simulink model "LW_ctrl_241029_1"  (R2024b)
settings: Solver=ode4  StartTime=0.0  StopTime=inf  FixedStep=0.005  RelTol=1e-3  EnableMultiTasking=on
StartFcn:
  | %timestart = cputime;
StopFcn:
  | %dt = cputime - timestart
undefined symbols (not defined in the file or in its folder): AttCtrl_cycle, ControlMode, DEG2RAD, Earth, FlightMode, LW_ACRO_P_MAX, LW_ACRO_R_MAX, LW_ACRO_Y_MAX, LW_AERO_C0, LW_AERO_C1, LW_AERO_Y0, LW_ANGLE, LW_DMZ0, LW_DMZ_MIN, LW_LAT_CIRCLE, LW_MAN_PITCH_MAX, LW_MAN_ROLL_MAX, LW_MASS, LW_OB_CIRCLE_R, LW_OB_CIRCLE_V, LW_OB_CIRCLE_W, LW_OB_TYPE, LW_REX_YAW, LW_SERVOL_MAX, LW_SERVOR_MAX, LW_TEST_DTXY, LW_TEST_DTZ, LW_THR_HOVER, LW_WZ_MAX, LW_X_ACCEL_MAX, LW_X_ACCEL_MIN, LW_X_FF, LW_X_JERK_MAX, LW_X_P, LW_X_VEL_MAX, LW_Y_ACCEL_MAX, LW_Y_ACCEL_MIN, LW_Y_FF, LW_Y_JERK_MAX, LW_Y_P, LW_Y_VEL_MAX, LW_YAW_KAD, LW_YAW_KAP, LW_Z_ACCEL_LOW, LW_Z_ACCEL_UP, LW_Z_FF, LW_Z_JERK_MAX, LW_Z_P, LW_Z_VEL_MAX_UP, Map_xoffset, Map_yoffset, Map_zoffset, MAX_wdotx, MAX_wdoty, MAX_wdotz, Mixer_cycle, ModelParam_AccelMax, ModelParam_DelayAtt, ModelParam_DelayOmega, ModelParam_DelayPos ... (+59)
libraries: pixhawk_slib_uORB_RW x15, simulink x7, slpidlib x6, dspfdesign x6, dspstat3 x5, aerolibnav x4, pixhawk_slib_sensors_actuators x3, aerolibtransform2 x3, etargetslib x2, pixhawk_slib_rfly x1, aerolibatmos2 x1, slrealtimeiplib x1
(part 6 of 6)

== matlab function LW_ctrl_241029_1/states_update/vehicle_local_position/HIL&FLY V1.13.3/DisturbanceEstimator ==
  data: Va input; qm input single; omegam input single; T input single; ModelParam_uavJ parameter; ModelParam_motorJm parameter; ModelParam_rotorEta parameter; ModelParam_rotordx parameter; ModelParam_rotordy parameter; ModelParam_rotorCm parameter; ModelParam_rotorCt parameter; qk_ output; omegak_ output; d_hat output single size=[3,1]; LW_TEST_WNXY parameter; LW_TEST_WNZ parameter; LW_TEST_LAMXY parameter; LW_TEST_LAMZ parameter; LW_TEST_SIGXY parameter; LW_TEST_SIGZ parameter; ModelParam_LBb parameter; ModelParam_LBc parameter; ModelParam_LBS parameter; LW_ANGLE parameter; ModelParam_LBRho parameter; LW_USE_SER parameter; LW_LBCL_D parameter; LW_LBCM_D parameter; ModelParam_LBCn_d parameter; LW_TEST_TDT parameter; quat_reset_counter input; delta_q_reset input; dt input single
function [qk_, omegak_, d_hat] = DisturbanceEstimator(Va, qm, omegam, T,...
    ModelParam_uavJ,ModelParam_motorJm, ModelParam_rotorEta, ModelParam_rotordx, ModelParam_rotordy, ModelParam_rotorCm, ModelParam_rotorCt,...
    LW_TEST_WNXY, LW_TEST_WNZ,LW_TEST_LAMXY, LW_TEST_LAMZ, LW_TEST_SIGXY, LW_TEST_SIGZ, ModelParam_LBb, ModelParam_LBc, ModelParam_LBS, LW_ANGLE, ...
    ModelParam_LBRho, LW_USE_SER, LW_LBCL_D, LW_LBCM_D, ModelParam_LBCn_d, LW_TEST_TDT, quat_reset_counter, delta_q_reset, dt)

persistent tau_qk tau_omegak tau_z3
persistent  quat_reset_counter_
if isempty(quat_reset_counter_)
    quat_reset_counter_ = quat_reset_counter;
end

if isInfNan(qm)
    qm = single([1;0;0;0]);
else
    %qm = qm/(sqrt(qm'*qm));
    %qm = quatnormalize(qm');
    qm = qm(:);
end
if isInfNan(omegam)
    omegam = single([0;0;0]);
else
    omegam = omegam(:);
end
if isInfNan(T)
    T = single([0;0;0;0;0;0]);
else
    T = T(:);
end
if dt < 0.001
    dt = single(0.001);
elseif dt > 0.02
    dt = single(0.02);
end

if isempty(tau_qk)
    if notInfNan(qm)
        tau_qk = qm;
    else
        tau_qk = single([1;0;0;0]);
    end
end
if isInfNan(tau_qk)
    if notInfNan(qm)
        tau_qk = qm;
    else
        tau_qk = single([1;0;0;0]);
    end
end
if isempty(tau_omegak)
    if notInfNan(omegam)
        tau_omegak = omegam;
    else
        tau_omegak = single([0;0;0]);
    end
end
if isInfNan(tau_omegak)
    if notInfNan(omegam)
        tau_omegak = omegam;
    else
        tau_omegak = single([0;0;0]);
    end
end
if isempty(tau_z3)
    tau_z3 = single([0;0;0]);
end
if isInfNan(tau_z3)
    tau_z3 = single([0;0;0]);
end



%结构参数
rotorEta = single(ModelParam_rotorEta);
rotordx = single(ModelParam_rotordx);
rotordy = single(ModelParam_rotordy);
LBb = single(ModelParam_LBb);
LBc = single(ModelParam_LBc);
LBS = single(ModelParam_LBS);
kappa = single(LW_ANGLE*pi/180);
Rho = single(ModelParam_LBRho);
%动力系统参数
rotorCm = single(ModelParam_rotorCm);
rotorCt = single(ModelParam_rotorCt);
km_f = rotorCm/rotorCt;
Cl_d = single(LW_LBCL_D);
Cm_d = single(LW_LBCM_D);
Cn_d = single(ModelParam_LBCn_d);
%
Va_ = max(Va,0.1);
if LW_USE_SER > 0.5
    Q = 0.5*Rho*Va_^2*LBS;
else
    Q = single(0);
end
%滤波器参数
L = eye(3,2,"single");
wn = [LW_TEST_WNXY;LW_TEST_WNXY;LW_TEST_WNZ];%rad/s
sigma = [LW_TEST_SIGXY;LW_TEST_SIGXY;LW_TEST_SIGZ];
L(:,1) = wn.^2;
L(:,2) = 2*sigma.*wn;
lamda = single([LW_TEST_LAMXY;LW_TEST_LAMXY;LW_TEST_LAMZ]);
%滤波器结构
%reset处理
if quat_reset_counter_ ~= quat_reset_counter
    tau_q = quatmultiply(delta_q_reset(:)',tau_qk');
    tau_qk = tau_q';
    quat_reset_counter_ = quat_reset_counter;
end
q_err = quatmultiply(quatconj(tau_qk'), qm');
q_err = quatnormalize(q_err);
eta = constrain(q_err(1), single(-1), single(1));
epsilon = q_err(2 : 4);
theta = 2 * acos(eta);
theta = wrap_pi(theta);
if abs(theta) < 0.0873 % 5*pi/180
    Xi_e = sign(eta) * 2 * epsilon;
else
    Xi_e = sign(eta) / sin(theta / 2) * theta * epsilon;
end
e_q = Xi_e(:);
e_omega = omegam - tau_omegak;

%inv_uavJ = eye(3,3)/ModelParam_uavJ;
inv_uavJ = eye(3);
for ii = 1:3
    inv_uavJ(ii,ii) = 1/(ModelParam_uavJ(ii,ii));
end
%le = l1*eq+l2*ew
Le = L(:,1).*e_q + L(:,2).*e_omega;
K1 = km_f;
coseta = cos(rotorEta);
K2 = rotordy*coseta;
dxcoseta = rotordx*coseta;
%估计螺旋桨推力，根据混控器输出滤波得到
T = LowPass(T, LW_TEST_TDT);
B = [-K2       -K2        K2       K2      -Q*LBb*Cl_d*cos(kappa) Q*LBb*Cl_d*cos(kappa);
     dxcoseta  -dxcoseta dxcoseta -dxcoseta Q*LBc*Cm_d Q*LBc*Cm_d;
     K1        -K1       -K1      K1      Q*LBb*Cl_d*sin(kappa) -Q*LBb*Cl_d*sin(kappa)];
z3_ = tau_z3 + lamda.*Le*dt;
if LW_USE_SER > 0.5
    Fr = B*T;
else
    Fr = B(:,1:4)*T(1:4);
end

omegak_ = tau_omegak +(Le + z3_ + inv_uavJ*Fr- inv_uavJ*(cross(omegam,ModelParam_uavJ*omegam)))*dt;
delta_theta = [0 -omegak_(1) -omegak_(2) -omegak_(3);
               omegak_(1) 0 omegak_(3) -omegak_(2);
               omegak_(2) -omegak_(3) 0 omegak_(1);
               omegak_(3) omegak_(2) -omegak_(1) 0]*dt;
qk_ = (eye(4) + delta_theta/2)*tau_qk;
qk_ = qk_/(sqrt(qk_'*qk_));
d_hat = ModelParam_uavJ*(Le + z3_);

if notInfNan(z3_) && notInfNan(omegak_) && notInfNan(qk_)
    tau_z3 = z3_;
    tau_omegak = omegak_;
    tau_qk = qk_;
else
    tau_z3 = single([0;0;0]);
    tau_omegak = omegam;
    tau_qk = qm;
end

end

function d_est = LowPass(d_est,DT)
% DT = dt/(dt + Ts)
% 其中dt是采样周期，Ts是低通滤波器的时间常数
% 截止频率f = 1/Ts/2pi Hz
% 如 dt=0.004, f=30Hz , LW_TEST_DT=0.43
persistent d_est_last
if isempty(d_est_last)
    d_est_last = d_est;
end
if isInfNan(d_est_last)
    d_est_last = zeros(size(d_est),'single');
end
d_est = d_est_last + DT*(d_est - d_est_last);
d_est_last = d_est;
end

== matlab function LW_ctrl_241029_1/rc_receive/manual_ctrl_in/Sim/Simulate RC/InputConditioning/deadzone1 ==
  data: u input; y output; rc_min input; rc_max input
function y = fcn(u, rc_min, rc_max)
%Function description:
%  Control the range of the remote control input from RCMin to RCMax, and set
%  a dead zone with a dead zone size of ±deadZone,the output y is
%  normalized to 0~1.You can get the RC calibration parameters in QGC.
RCMin = rc_min;
RCMax = rc_max;
RCMid = ((RCMin + RCMax)/2);
deadZoneRate = double(0.05);
deadZone = deadZoneRate*(RCMax - RCMin);
k = 1/(RCMax - RCMid - deadZone);
%Limiting
if(u < RCMin)
    u = RCMin;
elseif(u > RCMax)
    u = RCMax;
end
%dead zone and normalize
 if(u > RCMid + deadZone)
    y = single((u-RCMid - deadZone)*k);
 elseif(u < RCMid - deadZone)
     y = single((u - RCMid + deadZone)*k);
 else
     y = single(0);
 end
 end

== matlab function LW_ctrl_241029_1/navigator/logger/HIL&FLY/hrt_timestamp ==
  data: ts output
function ts  = fcn
% coder.cinclude('drivers/drv_hrt.h');
persistent count
if isempty(count)
    count = 0;
end

hrt = 0;
if coder.target('Rtw')
    hrt = coder.ceval('hrt_absolute_time');
else
    hrt = count;
end
ts = hrt;% us

count = count + 1;

== matlab function LW_ctrl_241029_1/rc_receive/manual_ctrl_in/Sim/Simulate RC/InputConditioning/deadzone2 ==
  data: u input; y output; rc_min input; rc_max input
function y = fcn(u, rc_min, rc_max)
%Function description:
%  Control the range of the remote control input from RCMin to RCMax, and set
%  a dead zone with a dead zone size of ±deadZone,the output y is
%  normalized to 0~1.You can get the RC calibration parameters in QGC.
RCMin = rc_min;
RCMax = rc_max;
RCMid = ((RCMin + RCMax)/2);
deadZoneRate = double(0.05);
deadZone = deadZoneRate*(RCMax - RCMin);
k = 1/(RCMax - RCMid - deadZone);
%Limiting
if(u < RCMin)
    u = RCMin;
elseif(u > RCMax)
    u = RCMax;
end
%dead zone and normalize
 if(u > RCMid + deadZone)
    y = single((u-RCMid - deadZone)*k);
 elseif(u < RCMid - deadZone)
     y = single((u - RCMid + deadZone)*k);
 else
     y = single(0);
 end
 end

== matlab function LW_ctrl_241029_1/state_machine/logger/HIL&FLY/hrt_timestamp ==
  data: ts output
function ts  = fcn
% coder.cinclude('drivers/drv_hrt.h');
persistent count
if isempty(count)
    count = 0;
end

hrt = 0;
if coder.target('Rtw')
    hrt = coder.ceval('hrt_absolute_time');
else
    hrt = count;
end
ts = hrt;% us

count = count + 1;

== matlab function LW_ctrl_241029_1/rc_receive/manual_ctrl_in/HIL&FLY V1.13.3/logger/hrt_timestamp ==
  data: ts output
function ts  = fcn
% coder.cinclude('drivers/drv_hrt.h');
persistent count
if isempty(count)
    count = 0;
end

hrt = 0;
if coder.target('Rtw')
    hrt = coder.ceval('hrt_absolute_time');
else
    hrt = count;
end
ts = hrt;% us

count = count + 1;

== matlab function LW_ctrl_241029_1/rc_receive/manual_ctrl_in/Sim/Simulate RC/InputConditioning/deadzone3 ==
  data: u input; y output; rc_min input; rc_max input
function y = fcn(u, rc_min, rc_max)
%Function description:
%  Control the range of the remote control input from RCMin to RCMax, and set
%  a dead zone with a dead zone size of ±deadZone,the output y is
%  normalized to 0~1.You can get the RC calibration parameters in QGC.
RCMin = rc_min;
RCMax = rc_max;
RCMid = ((RCMin + RCMax)/2);
deadZoneRate = double(0.05);
deadZone = deadZoneRate*(RCMax - RCMin);
k = 1/(RCMax - RCMid - deadZone);
%Limiting
if(u < RCMin)
    u = RCMin;
elseif(u > RCMax)
    u = RCMax;
end
%dead zone and normalize
 if(u > RCMid + deadZone)
    y = single((u-RCMid - deadZone)*k);
 elseif(u < RCMid - deadZone)
     y = single((u - RCMid + deadZone)*k);
 else
     y = single(0);
 end
 end

== matlab function LW_ctrl_241029_1/states_update/vehicle_local_position/Sim/nan_inf_q ==
  data: u input; y output
function y = fcn(u)

for i = 1:length(u)
    if isnan(u(i)) || isinf(u(i))
        if i == 1
            u(i) = single(1);
        else
            u(i) = single(0);
        end
    end
end
y = u;

== matlab function LW_ctrl_241029_1/navigator/navigator_manual/roll_deadzone ==
  data: u input; y output; LW_MAN_ROLL_DZ parameter
function y = fcn(u, LW_MAN_ROLL_DZ)
%Function description:
%  set a dead zone with a dead zone size of ±deadZone.
RCMin = single(-1);
RCMax = single(1);
RCMid = ((RCMin + RCMax)/2);
deadZone = LW_MAN_ROLL_DZ;
k = 1/(RCMax - RCMid - deadZone);

%dead zone
if(u > RCMid + deadZone)
    y = single((u-RCMid - deadZone)*k);
elseif(u < RCMid - deadZone)
    y = single((u - RCMid + deadZone)*k);
else
    y = single(0);
end
end

== matlab function LW_ctrl_241029_1/navigator/navigator_manual/pitch_deadzone ==
  data: u input; y output; LW_MAN_PITCH_DZ parameter
function y = fcn(u, LW_MAN_PITCH_DZ)
%Function description:
%  set a dead zone with a dead zone size of ±deadZone.
RCMin = single(-1);
RCMax = single(1);
RCMid = ((RCMin + RCMax)/2);
deadZone = LW_MAN_PITCH_DZ;
k = 1/(RCMax - RCMid - deadZone);

%dead zone
if(u > RCMid + deadZone)
    y = single((u-RCMid - deadZone)*k);
elseif(u < RCMid - deadZone)
    y = single((u - RCMid + deadZone)*k);
else
    y = single(0);
end
end

== matlab function LW_ctrl_241029_1/navigator/navigator_manual/rollrate_deadzone ==
  data: u input; y output; LW_MAN_WX_DZ parameter
function y = fcn(u, LW_MAN_WX_DZ)
%Function description:
%  set a dead zone with a dead zone size of ±deadZone.
RCMin = single(-1);
RCMax = single(1);
RCMid = ((RCMin + RCMax)/2);
deadZone = LW_MAN_WX_DZ;
k = 1/(RCMax - RCMid - deadZone);

%dead zone
if(u > RCMid + deadZone)
    y = single((u-RCMid - deadZone)*k);
elseif(u < RCMid - deadZone)
    y = single((u - RCMid + deadZone)*k);
else
    y = single(0);
end
end

== matlab function LW_ctrl_241029_1/navigator/navigator_manual/pitchrate_deadzone ==
  data: u input; y output; LW_MAN_WY_DZ parameter
function y = fcn(u, LW_MAN_WY_DZ)
%Function description:
%  set a dead zone with a dead zone size of ±deadZone.
RCMin = single(-1);
RCMax = single(1);
RCMid = ((RCMin + RCMax)/2);
deadZone = LW_MAN_WY_DZ;
k = 1/(RCMax - RCMid - deadZone);

%dead zone
if(u > RCMid + deadZone)
    y = single((u-RCMid - deadZone)*k);
elseif(u < RCMid - deadZone)
    y = single((u - RCMid + deadZone)*k);
else
    y = single(0);
end
end

== matlab function LW_ctrl_241029_1/navigator/navigator_manual/yawrate_deadzone ==
  data: u input; y output; LW_MAN_WZ_DZ parameter
function y = fcn(u, LW_MAN_WZ_DZ)
%Function description:
%  set a dead zone with a dead zone size of ±deadZone.
RCMin = single(-1);
RCMax = single(1);
RCMid = ((RCMin + RCMax)/2);
deadZone = LW_MAN_WZ_DZ;
k = 1/(RCMax - RCMid - deadZone);

%dead zone
if(u > RCMid + deadZone)
    y = single((u-RCMid - deadZone)*k);
elseif(u < RCMid - deadZone)
    y = single((u - RCMid + deadZone)*k);
else
    y = single(0);
end
end

== matlab function LW_ctrl_241029_1/navigator/navigator_manual/vx_deadzone ==
  data: u input; y output; LW_X_VEL_DZ parameter
function y = fcn(u, LW_X_VEL_DZ)
%Function description:
%  set a dead zone with a dead zone size of ±deadZone.
RCMin = single(-1);
RCMax = single(1);
RCMid = ((RCMin + RCMax)/2);
deadZone = LW_X_VEL_DZ;
k = 1/(RCMax - RCMid - deadZone);

%dead zone
if(u > RCMid + deadZone)
    y = single((u-RCMid - deadZone)*k);
elseif(u < RCMid - deadZone)
    y = single((u - RCMid + deadZone)*k);
else
    y = single(0);
end
end

== matlab function LW_ctrl_241029_1/navigator/navigator_manual/vy_deadzone ==
  data: u input; y output; LW_Y_VEL_DZ parameter
function y = fcn(u, LW_Y_VEL_DZ)
%Function description:
%  set a dead zone with a dead zone size of ±deadZone.
RCMin = single(-1);
RCMax = single(1);
RCMid = ((RCMin + RCMax)/2);
deadZone = LW_Y_VEL_DZ;
k = 1/(RCMax - RCMid - deadZone);

%dead zone
if(u > RCMid + deadZone)
    y = single((u-RCMid - deadZone)*k);
elseif(u < RCMid - deadZone)
    y = single((u - RCMid + deadZone)*k);
else
    y = single(0);
end
end

== matlab function LW_ctrl_241029_1/navigator/navigator_manual/vz_deadzone ==
  data: u input; y output; LW_Z_VEL_DZ parameter
function y = fcn(u, LW_Z_VEL_DZ)
%Function description:
%  set a dead zone with a dead zone size of ±deadZone.
% u:0-1
u = u*2 - 1; % -1~1
RCMin = single(-1);
RCMax = single(1);
RCMid = ((RCMin + RCMax)/2);
deadZone = LW_Z_VEL_DZ;
k = 1/(RCMax - RCMid - deadZone);

%dead zone
if(u > RCMid + deadZone)
    y = single((u-RCMid - deadZone)*k);
elseif(u < RCMid - deadZone)
    y = single((u - RCMid + deadZone)*k);
else
    y = single(0);
end
end

== matlab function LW_ctrl_241029_1/rc_receive/manual_ctrl_in/Sim/Simulate ref/commandMapping/command2pwm/stabilized/roll_deadzone_inv ==
  data: u input; y output; LW_MAN_ROLL_DZ parameter
function y = fcn(u, LW_MAN_ROLL_DZ)
%Function description:
%  set a dead zone with a dead zone size of ±deadZone.
RCMin = single(-1);
RCMax = single(1);
RCMid = ((RCMin + RCMax)/2);
deadZone = LW_MAN_ROLL_DZ;
k = 1/(RCMax - RCMid - deadZone);

%dead zone
if(u > RCMid + deadZone)
    y = single(u/k + RCMid + deadZone);
elseif(u < RCMid - deadZone)
     y = single(u/k + RCMid - deadZone);
else
    y = single(0);
end
end

== matlab function LW_ctrl_241029_1/rc_receive/manual_ctrl_in/Sim/Simulate ref/commandMapping/command2pwm/stabilized/pitch_deadzone_inv ==
  data: u input; y output; LW_MAN_PITCH_DZ parameter
function y = fcn(u, LW_MAN_PITCH_DZ)
%Function description:
%  set a dead zone with a dead zone size of ±deadZone.
RCMin = single(-1);
RCMax = single(1);
RCMid = ((RCMin + RCMax)/2);
deadZone = LW_MAN_PITCH_DZ;
k = 1/(RCMax - RCMid - deadZone);

%dead zone
if(u > RCMid + deadZone)
    y = single(u/k + RCMid + deadZone);
elseif(u < RCMid - deadZone)
     y = single(u/k + RCMid - deadZone);
else
    y = single(0);
end
end

== matlab function LW_ctrl_241029_1/rc_receive/manual_ctrl_in/Sim/Simulate ref/commandMapping/command2pwm/stabilized/yawrare_deadzone_inv ==
  data: u input; y output; LW_MAN_WZ_DZ parameter
function y = fcn(u, LW_MAN_WZ_DZ)
%Function description:
%  set a dead zone with a dead zone size of ±deadZone.
RCMin = single(-1);
RCMax = single(1);
RCMid = ((RCMin + RCMax)/2);
deadZone = LW_MAN_WZ_DZ;
k = 1/(RCMax - RCMid - deadZone);

%dead zone
if(u > RCMid + deadZone)
    y = single(u/k + RCMid + deadZone);
elseif(u < RCMid - deadZone)
     y = single(u/k + RCMid - deadZone);
else
    y = single(0);
end
end

== matlab function LW_ctrl_241029_1/rc_receive/manual_ctrl_in/Sim/Simulate ref/commandMapping/command2pwm/altitude/pitch_deadzone_inv ==
  data: u input; y output; LW_MAN_PITCH_DZ parameter
function y = fcn(u, LW_MAN_PITCH_DZ)
%Function description:
%  set a dead zone with a dead zone size of ±deadZone.
RCMin = single(-1);
RCMax = single(1);
RCMid = ((RCMin + RCMax)/2);
deadZone = LW_MAN_PITCH_DZ;
k = 1/(RCMax - RCMid - deadZone);

%dead zone
if(u > RCMid + deadZone)
    y = single(u/k + RCMid + deadZone);
elseif(u < RCMid - deadZone)
     y = single(u/k + RCMid - deadZone);
else
    y = single(0);
end
end

== matlab function LW_ctrl_241029_1/rc_receive/manual_ctrl_in/Sim/Simulate ref/commandMapping/command2pwm/altitude/roll_deadzone_inv ==
  data: u input; y output; LW_MAN_ROLL_DZ parameter
function y = fcn(u, LW_MAN_ROLL_DZ)
%Function description:
%  set a dead zone with a dead zone size of ±deadZone.
RCMin = single(-1);
RCMax = single(1);
RCMid = ((RCMin + RCMax)/2);
deadZone = LW_MAN_ROLL_DZ;
k = 1/(RCMax - RCMid - deadZone);

%dead zone
if(u > RCMid + deadZone)
    y = single(u/k + RCMid + deadZone);
elseif(u < RCMid - deadZone)
     y = single(u/k + RCMid - deadZone);
else
    y = single(0);
end
end

== matlab function LW_ctrl_241029_1/rc_receive/manual_ctrl_in/Sim/Simulate ref/commandMapping/command2pwm/acro/wz_deadzone_inv ==
  data: u input; y output; LW_MAN_WZ_DZ parameter
function y = fcn(u, LW_MAN_WZ_DZ)
%Function description:
%  set a dead zone with a dead zone size of ±deadZone.
RCMin = single(-1);
RCMax = single(1);
RCMid = ((RCMin + RCMax)/2);
deadZone = LW_MAN_WZ_DZ;
k = 1/(RCMax - RCMid - deadZone);

%dead zone
if(u > RCMid + deadZone)
    y = single(u/k + RCMid + deadZone);
elseif(u < RCMid - deadZone)
     y = single(u/k + RCMid - deadZone);
else
    y = single(0);
end
end

== matlab function LW_ctrl_241029_1/rc_receive/manual_ctrl_in/Sim/Simulate ref/commandMapping/command2pwm/acro/wx_deadzone_inv ==
  data: u input; y output; LW_MAN_WX_DZ parameter
function y = fcn(u, LW_MAN_WX_DZ)
%Function description:
%  set a dead zone with a dead zone size of ±deadZone.
RCMin = single(-1);
RCMax = single(1);
RCMid = ((RCMin + RCMax)/2);
deadZone = LW_MAN_WX_DZ;
k = 1/(RCMax - RCMid - deadZone);

%dead zone
if(u > RCMid + deadZone)
    y = single(u/k + RCMid + deadZone);
elseif(u < RCMid - deadZone)
     y = single(u/k + RCMid - deadZone);
else
    y = single(0);
end
end

== matlab function LW_ctrl_241029_1/rc_receive/manual_ctrl_in/Sim/Simulate ref/commandMapping/command2pwm/acro/wy_deadzone_inv ==
  data: u input; y output; LW_MAN_WY_DZ parameter
function y = fcn(u, LW_MAN_WY_DZ)
%Function description:
%  set a dead zone with a dead zone size of ±deadZone.
RCMin = single(-1);
RCMax = single(1);
RCMid = ((RCMin + RCMax)/2);
deadZone = LW_MAN_WY_DZ;
k = 1/(RCMax - RCMid - deadZone);

%dead zone
if(u > RCMid + deadZone)
    y = single(u/k + RCMid + deadZone);
elseif(u < RCMid - deadZone)
     y = single(u/k + RCMid - deadZone);
else
    y = single(0);
end
end

== matlab function LW_ctrl_241029_1/rc_receive/manual_ctrl_in/Sim/Simulate ref/commandMapping/command2pwm/position/wz_deadzone_inv ==
  data: u input; y output; LW_MAN_WZ_DZ parameter
function y = fcn(u, LW_MAN_WZ_DZ)
%Function description:
%  set a dead zone with a dead zone size of ±deadZone.
RCMin = single(-1);
RCMax = single(1);
RCMid = ((RCMin + RCMax)/2);
deadZone = LW_MAN_WZ_DZ;
k = 1/(RCMax - RCMid - deadZone);

%dead zone
if(u > RCMid + deadZone)
    y = single(u/k + RCMid + deadZone);
elseif(u < RCMid - deadZone)
     y = single(u/k + RCMid - deadZone);
else
    y = single(0);
end
end

== matlab function LW_ctrl_241029_1/rc_receive/manual_ctrl_in/Sim/Simulate ref/commandMapping/command2pwm/position/vz_deadzone_inv ==
  data: u input; y output; LW_Z_VEL_DZ parameter
function y = fcn(u, LW_Z_VEL_DZ)
%Function description:
%  set a dead zone with a dead zone size of ±deadZone.
RCMin = single(-1);
RCMax = single(1);
RCMid = ((RCMin + RCMax)/2);
deadZone = LW_Z_VEL_DZ;
k = 1/(RCMax - RCMid - deadZone);

%dead zone
if(u > RCMid + deadZone)
    y = single(u/k + RCMid + deadZone);
elseif(u < RCMid - deadZone)
     y = single(u/k + RCMid - deadZone);
else
    y = single(0);
end

y = (y+1)*0.5;
end

== matlab function LW_ctrl_241029_1/rc_receive/manual_ctrl_in/Sim/Simulate ref/commandMapping/command2pwm/position/vy_deadzone_inv ==
  data: u input; y output; LW_Y_VEL_DZ parameter
function y = fcn(u, LW_Y_VEL_DZ)
%Function description:
%  set a dead zone with a dead zone size of ±deadZone.
RCMin = single(-1);
RCMax = single(1);
RCMid = ((RCMin + RCMax)/2);
deadZone = LW_Y_VEL_DZ;
k = 1/(RCMax - RCMid - deadZone);

%dead zone
if(u > RCMid + deadZone)
    y = single(u/k + RCMid + deadZone);
elseif(u < RCMid - deadZone)
     y = single(u/k + RCMid - deadZone);
else
    y = single(0);
end
end

== matlab function LW_ctrl_241029_1/rc_receive/manual_ctrl_in/Sim/Simulate ref/commandMapping/command2pwm/position/vx_deadzone_inv ==
  data: u input; y output; LW_X_VEL_DZ parameter
function y = fcn(u, LW_X_VEL_DZ)
%Function description:
%  set a dead zone with a dead zone size of ±deadZone.
RCMin = single(-1);
RCMax = single(1);
RCMid = ((RCMin + RCMax)/2);
deadZone = LW_X_VEL_DZ;
k = 1/(RCMax - RCMid - deadZone);

%dead zone
if(u > RCMid + deadZone)
    y = single(u/k + RCMid + deadZone);
elseif(u < RCMid - deadZone)
     y = single(u/k + RCMid - deadZone);
else
    y = single(0);
end
end

== matlab function LW_ctrl_241029_1/rc_receive/manual_ctrl_in/Sim/Simulate ref/commandMapping/command2pwm/altitude/vz_deadzone_inv ==
  data: u input; y output; LW_Z_VEL_DZ parameter
function y = fcn(u, LW_Z_VEL_DZ)
%Function description:
%  set a dead zone with a dead zone size of ±deadZone.
RCMin = single(-1);
RCMax = single(1);
RCMid = ((RCMin + RCMax)/2);
deadZone = LW_Z_VEL_DZ;
k = 1/(RCMax - RCMid - deadZone);

%dead zone
if(u > RCMid + deadZone)
    y = single(u/k + RCMid + deadZone);
elseif(u < RCMid - deadZone)
     y = single(u/k + RCMid - deadZone);
else
    y = single(0);
end

y = (y+1)*0.5;
end

== matlab function LW_ctrl_241029_1/rc_receive/manual_ctrl_in/Sim/Simulate ref/commandMapping/command2pwm/altitude/wz_deadzone_inv ==
  data: u input; y output; LW_MAN_WZ_DZ parameter
function y = fcn(u, LW_MAN_WZ_DZ)
%Function description:
%  set a dead zone with a dead zone size of ±deadZone.
RCMin = single(-1);
RCMax = single(1);
RCMid = ((RCMin + RCMax)/2);
deadZone = LW_MAN_WZ_DZ;
k = 1/(RCMax - RCMid - deadZone);

%dead zone
if(u > RCMid + deadZone)
    y = single(u/k + RCMid + deadZone);
elseif(u < RCMid - deadZone)
     y = single(u/k + RCMid - deadZone);
else
    y = single(0);
end
end

== matlab function LW_ctrl_241029_1/states_update/vehicle_local_position/Sim/getIncid ==
  data: q input; incid output; LW_ANGLE parameter
function incid = fcn(q, LW_ANGLE)

if notInfNan(q)
    euler = my_quat2eul(q);
else
    euler = single([0;0;0]);
end
theta = euler(2);
alpha = theta + LW_ANGLE*pi/180;
beta = single(0);
incid = [alpha; beta];

== matlab function LW_ctrl_241029_1/navigator/navigator_manual/Lowpass ==
  data: data_in input; data_in output; LW_VEL_DT parameter
function data_in = fcn(data_in, LW_VEL_DT)
persistent data_last
if isempty(data_last)
    data_last = data_in;
end
if isInfNan(data_last)
    data_last = single(0);
end

data_in = data_last + LW_VEL_DT*(data_in - data_last);
data_last = data_in;

== matlab function LW_ctrl_241029_1/navigator/navigator_manual/Lowpass1 ==
  data: data_in input; data_in output; LW_VEL_DT parameter
function data_in = fcn(data_in, LW_VEL_DT)
persistent data_last
if isempty(data_last)
    data_last = data_in;
end
if isInfNan(data_last)
    data_last = single(0);
end

data_in = data_last + LW_VEL_DT*(data_in - data_last);
data_last = data_in;

== matlab function LW_ctrl_241029_1/states_update/vehicle_local_position/Sim/Lowpass ==
  data: d_est input; d_est output; LW_TEST_DTXY parameter; LW_TEST_DTZ parameter
function d_est = fcn(d_est,LW_TEST_DTXY,LW_TEST_DTZ)
% LW_TEST_DT = dt/(dt + Ts)
% 其中dt是采样周期，Ts是低通滤波器的时间常数
% 截止频率f = 1/Ts/2pi Hz
% 如 dt=0.004, f=30Hz , LW_TEST_DT=0.43
persistent d_est_last
if isempty(d_est_last)
    d_est_last = d_est;
end
if isInfNan(d_est_last)
    d_est_last = single([0;0;0]);
end
d_est(1:2) = d_est_last(1:2) + LW_TEST_DTXY*(d_est(1:2) - d_est_last(1:2));
d_est(3) = d_est_last(3) + LW_TEST_DTZ*(d_est(3) - d_est_last(3));

d_est_last = d_est;
end

== matlab function LW_ctrl_241029_1/Output/OutputSelect/Sim/Lifting Body Airframe/Estimator/Sensor Model/GPS/GenCogVel ==
  data: v output; u input; cot output
function [v,cot] = Ang360(u)
v=norm(u(1:2));

if v < 1
    cot = 0;
else
    cot=atan2d(u(2),u(1));
end
 
if cot<0
    cot=cot+360;
end

== matlab function LW_ctrl_241029_1/states_update/vehicle_local_position/HIL&FLY V1.13.3/Lowpass ==
  data: d_est input; d_est output; LW_TEST_DTXY parameter; LW_TEST_DTZ parameter
function d_est = fcn(d_est,LW_TEST_DTXY,LW_TEST_DTZ)
% LW_TEST_DT = dt/(dt + Ts)
% 其中dt是采样周期，Ts是低通滤波器的时间常数
% 截止频率f = 1/Ts/2pi Hz
% 如 dt=0.004, f=30Hz , LW_TEST_DT=0.43
persistent d_est_last
if isempty(d_est_last)
    d_est_last = d_est;
end
if isInfNan(d_est_last)
    d_est_last = single([0;0;0]);
end
d_est(1:2) = d_est_last(1:2) + LW_TEST_DTXY*(d_est(1:2) - d_est_last(1:2));
d_est(3) = d_est_last(3) + LW_TEST_DTZ*(d_est(3) - d_est_last(3));

d_est_last = d_est;
end

== matlab function LW_ctrl_241029_1/navigator/logger/Sim/quat2eul ==
  data: q input; euler output
function euler = fcn(q)
q = single(q);
euler = my_quat2eul(q,'ZYX');

== matlab function LW_ctrl_241029_1/Output/OutputSelect/Sim/Lifting Body Airframe/Estimator/Sensor Model/Magnetometer Hub/MATLAB Function ==
  data: DCM input; mag_e input; b_m input; n_m input; Mag_means output; K_m input
function Mag_means = fcn(DCM, mag_e, b_m, n_m, K_m)
 
Mag_means = K_m*DCM*mag_e + b_m + n_m;

== matlab function LW_ctrl_241029_1/Output/OutputSelect/Sim/Lifting Body Airframe/Estimator/Sensor Model/Magnetometer Hub/MATLAB Function1 ==
  data: DCM input; mag_e input; b_m input; n_m input; Mag_means output; K_m input
function Mag_means = fcn(DCM, mag_e, b_m, n_m, K_m)
 
Mag_means = K_m*DCM*mag_e + b_m + n_m;

== matlab function LW_ctrl_241029_1/Output/OutputSelect/Sim/Lifting Body Airframe/Estimator/Subsystem1/Quaternion to rotation matrix ==
  data: q input; Reb output
function Reb = fcn(q)
%Function description;
%  The rotation matrix of the body coordinate system to the geodetic coordinate system is obtained from the quaternion
Reb = [q(1)*q(1) + q(2)*q(2) - q(3)*q(3) - q(4)*q(4), 2*(q(2)*q(3) - q(1)*q(4)), 2*(q(2)*q(4) + q(1)*q(3))
       2*(q(2)*q(3) + q(1)*q(4)), q(1)*q(1) - q(2)*q(2) + q(3)*q(3) - q(4)*q(4), 2*(q(3)*q(4) - q(1)*q(2))
       2*(q(2)*q(4) - q(1)*q(3)), 2*(q(3)*q(4) + q(1)*q(2)), q(1)*q(1) - q(2)*q(2) - q(3)*q(3) + q(4)*q(4)];

== matlab function LW_ctrl_241029_1/Output/OutputSelect/Sim/Lifting Body Airframe/Estimator/Subsystem1/attitude_estimator ==
  data: dt input; phi_cf output; z input; phi_cf_k input; theta_cf_k input; tao input; theta_cf output
function [ phi_cf, theta_cf ] = Attitude_cf(dt, z, phi_cf_k, theta_cf_k, tao)
%Function description:
%  complementary filter  for attitude estimation.
%Input:
%  dt: sampling time, unit: s
%  z: three-axis gyroscope and three-axis accelerometer data, [gx, gy, gz, ax, ay, az]', unit: rad/s, m/s2
%  phi_cf_k, theta_cf_k: angle value of the previous sampling, unit: rad
%  tao: filter coefficient
%Output:
%  phi_cf, theta_cf: attitude angle, unit: rad
    persistent z_valid theta_cf_k_valid phi_cf_k_valid
    if isempty(z_valid)
        z_valid = zeros(6,1);
        theta_cf_k_valid = 0;
        phi_cf_k_valid = 0;
    end
    for i = 1:length(z)
    if isnan(z(i)) || isinf(z(i))
        z(i) = z_valid(i);
    else
        z_valid(i) = z(i);
    end
    end
     if isnan(theta_cf_k) || isinf(theta_cf_k)
        theta_cf_k = theta_cf_k_valid;
     else
         theta_cf_k_valid = theta_cf_k;
    end
    if isnan(phi_cf_k) || isinf(phi_cf_k)
        phi_cf_k = phi_cf_k_valid;
    else
        phi_cf_k_valid = phi_cf_k;
    end
    
    gx = z(1); gy = z(2);
    ax = z(4); ay = z(5); az = z(6);
    
    % calculate Euler angles using accelerometer data
    g = sqrt(ax*ax + ay*ay + az*az);
    if g < 9.8*0.95 || g > 9.8*1.05
        tao = 10000.0;
    end
    theta_am = asin(ax/g);
    phi_am = -asin(ay/(g*cos(theta_am)));
    
    
    % complementary filtering
    theta_cf = tao/(tao + dt)*(theta_cf_k + gy*dt) + dt/(tao + dt)*theta_am;
    phi_cf = tao/(tao + dt)*(phi_cf_k + gx*dt) + dt/(tao + dt)*phi_am;
end

== matlab function LW_ctrl_241029_1/Output/OutputSelect/Sim/Lifting Body Airframe/Estimator/Subsystem1/attitude_estimator1 ==
  data: dt input; x_aposteriori output; z input; q input; r input; x_aposteriori_k input; P_aposteriori output; P_aposteriori_k input; phi output; theta output
function [ x_aposteriori, P_aposteriori, phi, theta] = Attitude_ekf( dt, z, q, r, x_aposteriori_k, P_aposteriori_k)
%Function description:
%  Extended Kalman Filter for State Estimation
%Input:
%  dt: sampling time
%  z: measurement data (6,1)
%  q: system noise, r: measurement noise
%  x_aposteriori_k: estimated state at the last moment (6,1)
%  P_aposteriori_k: error covariance at the last moment (6,6)
%Output:
%  x_aposteriori：estimated state at current time (6,1)
%  P_aposteriori：error covariance at the current moment (6,6)
%  roll、pitch：Euler angle, unit: rad

 persistent z_valid x_aposteriori_k_valid P_aposteriori_k_valid
    if isempty(z_valid)
        z_valid = zeros(6,1);
        x_aposteriori_k_valid = [0, 0, 0, 0, 0, -1];
        P_aposteriori_k_valid = eye(6, 6)*100;
    end
    for i = 1:length(z)
    if isnan(z(i)) || isinf(z(i))
        z(i) = z_valid(i);
    else
        z_valid(i) = z(i);
    end
    end
     for i = 1:length(x_aposteriori_k)
    if isnan(x_aposteriori_k(i)) || isinf(x_aposteriori_k(i))
        x_aposteriori_k(i) = x_aposteriori_k_valid(i);
    else
        x_aposteriori_k_valid(i) = x_aposteriori_k(i);
    end
     end
     for i = 1:length(P_aposteriori_k)
     if isnan(P_aposteriori_k(i)) || isinf(P_aposteriori_k(i))
        P_aposteriori_k(i) = P_aposteriori_k_valid(i);
    else
        P_aposteriori_k_valid(i) = P_aposteriori_k(i);
     end
     end
   


w_m = z(1:3);  % angular velocity measurement
a_m = z(4:6);  % acceleration measurement
g = norm(a_m,2);   % gravitational acceleration
%   w_x_=[ 0,-(wz-bzg, wy-byg;
%         wz-bzg, 0 ,-(wx-bxg);
%         -(wy-byg), wx-bxg, 0];
w_x_ = [0, -(w_m(3) - x_aposteriori_k(3)), w_m(2) - x_aposteriori_k(2);
      w_m(3) - x_aposteriori_k(3), 0, -(w_m(1) - x_aposteriori_k(1));
      -(w_m(2) - x_aposteriori_k(2)), w_m(1) - x_aposteriori_k(1), 0];
     
bCn = eye(3, 3) - w_x_*dt;

%% predict
% update a priori state matrix
  x_apriori = zeros(1, 6);
  x_apriori(1: 3) = x_aposteriori_k(1 : 3);  % angular velocity drift
  x_apriori(4 : 6) = bCn*x_aposteriori_k(4 : 6);   % normalized acceleration
  
%[x]x
  x_aposteriori_k_x = [0, -x_aposteriori_k(6), x_aposteriori_k(5);
                        x_aposteriori_k(6), 0, -x_aposteriori_k(4);
                        -x_aposteriori_k(5), x_aposteriori_k(4), 0];
% update state transition matrix
PHI = [eye(3, 3), zeros(3, 3);
         -x_aposteriori_k_x*dt, bCn];
GAMMA = [eye(3, 3)*dt, zeros(3, 3);
       zeros(3, 3), -x_aposteriori_k_x*dt];

Q = [eye(3, 3)*q(1), zeros(3, 3);
   zeros(3, 3), eye(3, 3)*q(2)];
 % prediction error covariance matrix
 P_apriori = PHI*P_aposteriori_k*PHI' + GAMMA*Q*GAMMA';
%% update
 R = eye(3, 3)*r(1);
 H_k = [zeros(3, 3), -g*eye(3, 3)];
 % Kalman gain
 K_k = (P_apriori*H_k')/(H_k*P_apriori*H_k' + R);
  % state estimate update
 x_aposteriori = x_apriori' + K_k*(a_m - H_k*x_apriori');
 % error covariance update
 P_aposteriori = (eye(6, 6) - K_k*H_k)*P_apriori;
  %% calculate roll, pitch
  k = x_aposteriori(4 : 6) /norm(x_aposteriori(4 : 6), 2);
  
  phi = atan2(k(2), k(3));
  theta = -asin(k(1));
end

== matlab function LW_ctrl_241029_1/Output/OutputSelect/Sim/Lifting Body Airframe/Estimator/Subsystem1/euler2quad ==
  data: euler input; q output
function q = euler2quad(euler)
 %Function description;
%  Euler to Quaternion
%  euler = [phi, theta, psi];
euler = euler/2;
cphi = cos(euler(1)); sphi = sin(euler(1));
ctheta = cos(euler(2)); stheta = sin(euler(2));
cpsi = cos(euler(3)); spsi = sin(euler(3));
q = [cphi*ctheta*cpsi + sphi*stheta*spsi;
    sphi*ctheta*cpsi - cphi*stheta*spsi;
    cphi*stheta*cpsi + sphi*ctheta*spsi;
    cphi*ctheta*spsi - sphi*stheta*cpsi];

== matlab function LW_ctrl_241029_1/navigator/navigator_manual/nan_inf0 ==
  data: u input; y output
function y = fcn(u)

for i = 1:length(u)
    if isnan(u(i)) || isinf(u(i))
        u(i) = single(0);
    end
end
y = u;

== matlab function LW_ctrl_241029_1/navigator/navigator_manual/nan_inf1 ==
  data: u input; y output
function y = fcn(u)

for i = 1:length(u)
    if isnan(u(i)) || isinf(u(i))
        u(i) = single(0);
    end
end
y = u;

== matlab function LW_ctrl_241029_1/navigator/navigator_manual/nan_inf2 ==
  data: u input; y output
function y = fcn(u)

for i = 1:length(u)
    if isnan(u(i)) || isinf(u(i))
        u(i) = single(0);
    end
end
y = u;

== matlab function LW_ctrl_241029_1/navigator/navigator_manual/nan_inf3 ==
  data: u input; y output
function y = fcn(u)

for i = 1:length(u)
    if isnan(u(i)) || isinf(u(i))
        u(i) = single(0);
    end
end
y = u;

== matlab function LW_ctrl_241029_1/navigator/navigator_manual/nan_inf4 ==
  data: u input; y output
function y = fcn(u)

for i = 1:length(u)
    if isnan(u(i)) || isinf(u(i))
        u(i) = single(0);
    end
end
y = u;

== matlab function LW_ctrl_241029_1/navigator/navigator_manual/nan_inf5 ==
  data: u input; y output
function y = fcn(u)

for i = 1:length(u)
    if isnan(u(i)) || isinf(u(i))
        u(i) = single(0);
    end
end
y = u;

== matlab function LW_ctrl_241029_1/navigator/navigator_manual/nan_inf6 ==
  data: u input; y output
function y = fcn(u)

for i = 1:length(u)
    if isnan(u(i)) || isinf(u(i))
        u(i) = single(0);
    end
end
y = u;

== matlab function LW_ctrl_241029_1/navigator/navigator_manual/nan_inf7 ==
  data: u input; y output
function y = fcn(u)

for i = 1:length(u)
    if isnan(u(i)) || isinf(u(i))
        u(i) = single(0);
    end
end
y = u;

== matlab function LW_ctrl_241029_1/navigator/navigator_manual/nan_inf8 ==
  data: u input; y output
function y = fcn(u)

for i = 1:length(u)
    if isnan(u(i)) || isinf(u(i))
        u(i) = single(0);
    end
end
y = u;

== matlab function LW_ctrl_241029_1/rc_receive/manual_ctrl_in/Sim/Simulate ref/commandMapping/MATLAB Function ==
  data: flight_mode input; AU8 output
function AU8 = fcn(flight_mode)
if flight_mode == FlightMode.PILOT
    AU8 = 1000;
elseif flight_mode == FlightMode.AUTO
    AU8 = 1500;
else
    %offboard
    AU8 = 2000;
end

== matlab function LW_ctrl_241029_1/state_machine/MATLAB Function4 ==
  data: ctrl_mode output; ch5 input; ch7 input; ch8 input; flight_mode output; RC_Lost input; armed input
function [ctrl_mode, flight_mode]  = fcn(ch5, ch7, ch8, RC_Lost, armed)
%Function description:
%  Map the remote control CH5 channel to control mode
%input:
%  ch5: Remote control CH5 channel input
%  control_mode: Custom control mode
%  0: stablelize mode；1: height control mode; 2: position control mode
%  4: attitude rate mode
%  the remote control CH8 channel change the flight mode
%input:
%  ch8: Remote control CH8 channel input

if ch5 < 1400
    ctrl_mode = ControlMode.STABILIZED;
    if ch7 >1300 && ch7 < 1600
        %ctrl_mode = ControlMode.ACRO;
    elseif ch7 >= 1600
        ctrl_mode = ControlMode.MANUAL;
    end
elseif ch5 < 1600
    ctrl_mode = ControlMode.ALTITUDE;
else
    ctrl_mode = ControlMode.POSITION;
end
if ch8 < 1400
    flight_mode = FlightMode.PILOT;
% elseif ch8 < 1600
%     flight_mode = FlightMode.AUTO;
%     ctrl_mode = ControlMode.MISSION;
else
    flight_mode = FlightMode.OFFBOARD;
end

if RC_Lost > 0.5
%     flight_mode = FlightMode.AUTO;
%     ctrl_mode = ControlMode.LOITER;
end

% if armed > 0.5 && ch8 > 1500
%     flight_mode = FlightMode.OFFBOARD;
% end

== matlab function LW_ctrl_241029_1/Output/OutputSelect/Sim/Lifting Body Airframe/Estimator/nan_inf ==
  data: u input; y output
function y = fcn(u)

for i = 1:length(u)
    if isnan(u(i)) || isinf(u(i))
        u(i) = 0;
    end
end
y = u;

== matlab function LW_ctrl_241029_1/Output/OutputSelect/Sim/Lifting Body Airframe/Estimator/nan_inf1 ==
  data: u input; y output
function y = fcn(u)

for i = 1:length(u)
    if isnan(u(i)) || isinf(u(i))
        u(i) = 0;
    end
end
y = u;

== matlab function LW_ctrl_241029_1/navigator/navigator_manual/nan_inf10 ==
  data: u input; y output
function y = fcn(u)

for i = 1:length(u)
    if isnan(u(i)) || isinf(u(i))
        u(i) = single(0);
    end
end
y = u;

== matlab function LW_ctrl_241029_1/Output/OutputSelect/Sim/Lifting Body Airframe/Estimator/nan_inf2 ==
  data: u input; y output
function y = fcn(u)

for i = 1:length(u)
    if isnan(u(i)) || isinf(u(i))
        u(i) = 0;
    end
end
y = u;

== matlab function LW_ctrl_241029_1/Output/OutputSelect/Sim/Lifting Body Airframe/Estimator/nan_inf3 ==
  data: u input; y output
function y = fcn(u)

for i = 1:length(u)
    if isnan(u(i)) || isinf(u(i))
        u(i) = 0;
    end
end
y = u;

== matlab function LW_ctrl_241029_1/Output/OutputSelect/Sim/Lifting Body Airframe/Estimator/nan_inf4 ==
  data: u input; y output
function y = fcn(u)

for i = 1:length(u)
    if isnan(u(i)) || isinf(u(i))
        u(i) = 0;
    end
end
y = u;

== matlab function LW_ctrl_241029_1/Output/OutputSelect/Sim/Lifting Body Airframe/Estimator/nan_inf5 ==
  data: u input; y output
function y = fcn(u)

for i = 1:length(u)
    if isnan(u(i)) || isinf(u(i))
        u(i) = 0;
    end
end
y = u;

== matlab function LW_ctrl_241029_1/Output/OutputSelect/Sim/Lifting Body Airframe/Estimator/nan_inf6 ==
  data: u input; y output
function y = fcn(u)

for i = 1:length(u)
    if isnan(u(i)) || isinf(u(i))
        u(i) = 15;
    end
end
y = u;

== matlab function LW_ctrl_241029_1/Output/OutputSelect/Sim/Lifting Body Airframe/Estimator/nan_inf_q ==
  data: u input; y output
function y = fcn(u)

for i = 1:length(u)
    if isnan(u(i)) || isinf(u(i))
        if i == 1
            u(i) = 1;
        else
            u(i) = 0;
        end
    end
end
y = u;

== matlab function LW_ctrl_241029_1/Output/OutputSelect/Sim/Lifting Body Airframe/Get Terrain/getTerrainAltData ==
  settings: updateMethod=DISCRETE
  data: x input; z output; y input
function z = fcn(x,y)
%z=getTerrainAltData(x,y);
persistent zoffset
if isnan(x) || isnan(y)
   x = 0;
   y = 0;
end
if isempty(zoffset)
    zoffset = getTerrainAltData(x,y);
end
z=getTerrainAltData(x,y) - zoffset;

end

== matlab function LW_ctrl_241029_1/navigator/navigator_manual/Lowpass2 ==
  data: data_in input; data_in output; LW_VEL_DT parameter
function data_in = fcn(data_in, LW_VEL_DT)
persistent data_last
if isempty(data_last)
    data_last = data_in;
end
if isInfNan(data_last)
    data_last = single(0);
end

data_in = data_last + LW_VEL_DT*(data_in - data_last);
data_last = data_in;

== matlab function LW_ctrl_241029_1/states_update/vehicle_local_position/HIL&FLY V1.13.3/Lowpass1 ==
  data: d_est input; d_est output; LW_TEST_WBDT parameter
function d_est = fcn(d_est,LW_TEST_WBDT)
% LW_TEST_DT = dt/(dt + Ts)
% 其中dt是采样周期，Ts是低通滤波器的时间常数
% 截止频率f = 1/Ts/2pi Hz
% 如 dt=0.004, f=30Hz , LW_TEST_DT=0.43
persistent d_est_last
if isempty(d_est_last)
    d_est_last = d_est;
end
if isInfNan(d_est_last)
    d_est_last = single([0;0;0]);
end
d_est = d_est_last + LW_TEST_WBDT*(d_est - d_est_last);
d_est_last = d_est;
end

== matlab function LW_ctrl_241029_1/states_update/vehicle_local_position/Sim/Lowpass1 ==
  data: d_est input; d_est output; LW_TEST_WBDT parameter
function d_est = fcn(d_est,LW_TEST_WBDT)
% LW_TEST_DT = dt/(dt + Ts)
% 其中dt是采样周期，Ts是低通滤波器的时间常数
% 截止频率f = 1/Ts/2pi Hz
% 如 dt=0.004, f=30Hz , LW_TEST_DT=0.43
persistent d_est_last
if isempty(d_est_last)
    d_est_last = d_est;
end
if isInfNan(d_est_last)
    d_est_last = single([0;0;0]);
end
d_est = d_est_last + LW_TEST_WBDT*(d_est - d_est_last);
d_est_last = d_est;
end

== matlab function LW_ctrl_241029_1/navigator/navigator_offboard/task select/task select/task ==
  data: timestamp input; flight_mode input; pos input size=[3,1]; vel input size=[3,1]; q input; pos_ref output size=[3,1]; vel_ref output size=[3,1]; acc_ref output; euler_ref output; dot3x output; yaw_ref output; dotpsi output; LW_OB_CIRCLE_R parameter; LW_OB_CIRCLE_V parameter; LW_OB_CIRCLE_W parameter; LW_OB_TYPE parameter; reverse_flag output; CH8 input
function [pos_ref, vel_ref, acc_ref, euler_ref,dot3x, yaw_ref, dotpsi,reverse_flag] = fcn(timestamp, flight_mode,pos, vel, q, LW_OB_CIRCLE_R, LW_OB_CIRCLE_V, LW_OB_CIRCLE_W, LW_OB_TYPE,CH8)

if CH8 < 1600
    [pos_ref, vel_ref, acc_ref, euler_ref,dot3x, yaw_ref, dotpsi,reverse_flag] = task5(timestamp, flight_mode,pos, vel, q, LW_OB_CIRCLE_R, LW_OB_CIRCLE_V, LW_OB_CIRCLE_W, LW_OB_TYPE);
else
    [pos_ref, vel_ref, acc_ref, euler_ref,dot3x, yaw_ref, dotpsi,reverse_flag] = task1(timestamp, flight_mode,pos, vel, q, LW_OB_CIRCLE_R, LW_OB_CIRCLE_V, LW_OB_CIRCLE_W, LW_OB_TYPE);
end
end

== matlab function LW_ctrl_241029_1/navigator/navigator_offboard/task select/task select/df,coor,wind ==
  data: pos_ref input; vel_ref input; acc_ref input; euler_ref input; dot3x input; yaw_ref input; dotpsi input; v_wind input; pos_ref output; vel_ref output; acc_ref output; q_ref output; f_d output; alpha output; beta output; wb_ref output; dotwb_ref output; ModelParam_LBRho parameter; ModelParam_LBS parameter; ModelParam_pu_c0 parameter; ModelParam_pu_c1 parameter; LW_AERO_Y0 parameter; LW_ANGLE parameter; ModelParam_pu_c2 parameter; ModelParam_pu_c3 parameter; ModelParam_envGravityAcc parameter; LW_AERO_C0 parameter; LW_AERO_C1 parameter; LW_MASS parameter; OB_TASK output; eee output
function [pos_ref, vel_ref, acc_ref, q_ref, f_d, alpha,beta, wb_ref, dotwb_ref, OB_TASK,eee] = fcn(pos_ref, vel_ref, acc_ref, euler_ref, dot3x, yaw_ref, dotpsi, v_wind, ...
    ModelParam_LBRho, ModelParam_LBS, ModelParam_pu_c0, ModelParam_pu_c1, LW_AERO_Y0, LW_ANGLE, ModelParam_pu_c2, ModelParam_pu_c3, ModelParam_envGravityAcc, LW_AERO_C0, LW_AERO_C1, LW_MASS)

% Note
% adopt the results from differential Flatness derived from data 2022-6-16
% 加入风

persistent xw_  yb_
if isempty(xw_)
    if ~isnan(yaw_ref)
        xw_ = [cos(yaw_ref) sin(yaw_ref) 0]';
        yb_ = [-sin(yaw_ref) cos(yaw_ref) 0]';
    else
        xw_ = single([1 0 0]');
        yb_ = single([0 1 0]');
    end 
end
%% 
airspeed_T = single(0.01);
g = single([0; 0; ModelParam_envGravityAcc]);
Cd0 = single(ModelParam_pu_c0); % 最小阻力
Cla = single(ModelParam_pu_c1); % post stall
Cd0 = single(LW_AERO_C0); % 最小阻力
Cla = single(LW_AERO_C1); % post stall

% Cd0 = single(ModelParam_pu_c3); % 最小阻力
% Cla = single(ModelParam_pu_c2); % pre stall
Cy0 = single(LW_AERO_Y0);
kk = single(LW_ANGLE*pi/180);
Rho = single(ModelParam_LBRho);
Mass = single(LW_MASS);


dotdotx = single(acc_ref(:));
va = single(vel_ref(:) - v_wind);
Va = sqrt(va'*va);
Qa = 0.5/Mass * Rho * ModelParam_LBS * Va;

if ~isnan(yaw_ref)
    xw_ = [cos(yaw_ref) sin(yaw_ref) 0]';
    yb_ = [-sin(yaw_ref) cos(yaw_ref) 0]';
end

if Va > airspeed_T && isnan(yaw_ref)
    xw = va / Va;
    xw_ = xw;
else
    xw = xw_;
end

    a_xw = xw' * (dotdotx - g);
    an = dotdotx - g - a_xw * xw;
    a_zw = -norm(an);
    [f_d, alpha] = SolveFza(a_xw, a_zw, Va, Cd0, Cla, Rho,  ModelParam_LBS, LW_MASS, kk);

    ay = Qa * Cy0 * va - g + dotdotx;
    xw_ay_norm = norm(cross(xw, ay));
    if xw_ay_norm > 0.01
        yb = cross(xw, ay) / xw_ay_norm;
        yb_ = yb;
    else
        yb = yb_;
    end
    yb_hat = [0 -yb(3) yb(2); yb(3) 0 -yb(1); -yb(2) yb(1) 0];
    lamda = alpha - kk;
    xb = (cos(lamda)*eye(3) + (1 - cos(lamda))*yb*yb'+sin(lamda)*yb_hat)*xw;
    zb = cross(xb, yb);
    R_d = [xb yb zb];
    %协调假设求解角速度
    wb_ref = calculateWb(f_d, R_d, Va, va, dotdotx, dot3x, Cd0, Cla, Cy0, Rho, ModelParam_LBS, LW_MASS, g, kk);
    q_ref = R2quat(R_d);
    dotwb_ref = zeros(3,1,'single');
    beta = single(0);
    OB_TASK = int8(2);
    eee = my_quat2eul(q_ref);
end

function [fz, alpha] = SolveFza(av1_, av3_, Va, Cd0, Cla, Rho, S, m, kk)

Q = 0.5 * Rho * Va ^ 2;
QSCla = Q * S * Cla;

av1 = av1_*m + Q * S * Cd0;
av3 = min(av3_*m, 0);
k1 = sqrt(av1 ^ 2 * cos(kk) ^ 2 + (av1 + QSCla) ^ 2 * sin(kk) ^ 2 + av3 ^ 2 - QSCla * av3 * sin(2 * kk));
fz = -(av1^2 + QSCla*av1 + av3^2) / k1;

alpha = 2 * atan((QSCla * sin(kk) - av3 * cos(kk) + av1 * sin(kk) - k1) / (av1 * cos(kk) + av3 * sin(kk)));
end

function wbb = calculateWb(fz, Rbb, Vg, dotx, dotdotx, dot3x, Cd0, Cla, Cy0, Rho, S, m, g, kk)
    persistent wz_ wx_
    if isempty(wz_)
        wz_ = single(0);
        wx_ = single(0);
    end
    Qa = 0.5/m * Rho * S * Vg;
    cz = fz/m;
    dxz = Cla * sin(kk) * cos(kk);
    dx = Cd0 + Cla * sin(kk) ^ 2;
    dz = Cd0 + Cla * cos(kk) ^ 2;
    
    if Vg < 0.01
        C1 = Rbb(:, 1)' * dot3x + Qa * (dx * Rbb(:, 1)' * dotdotx + dxz * Rbb(:, 3)' * dotdotx);
    else
        C1 = Rbb(:, 1)' * dot3x + Qa*dotx'*dotdotx/(Vg^2)*(dx * Rbb(:, 1)' * dotx + dxz * Rbb(:, 3)' * dotx)+ Qa * (dx * Rbb(:, 1)' * dotdotx + dxz * Rbb(:, 3)' * dotdotx);
    end
    
    A1 = Qa * dxz * Rbb(:, 2)' * dotx;
    B1 = cz - Qa * ((dz - dx) * Rbb(:, 3)' * dotx + 2*dxz * Rbb(:, 1)' * dotx);
    D1 = -Qa * ((dx - Cy0) * Rbb(:, 2)' * dotx);
    if Vg < 0.01
        C2 = Rbb(:, 2)' * dot3x + Qa * Cy0 * Rbb(:, 2)' * dotdotx;
    else
        C2 = Rbb(:, 2)' * dot3x + Qa*dotx'*dotdotx/(Vg^2)*(Cy0 * Rbb(:, 2)' * dotx)+ Qa * Cy0 * Rbb(:, 2)' * dotdotx;
    end
    A2 = -cz + Qa * (dxz * Rbb(:, 1)' * dotx + (dz - Cy0) * Rbb(:, 3)' * dotx);
    D2 = -Qa * ((dx - Cy0) * Rbb(:, 1)' * dotx + dxz * Rbb(:, 3)' * dotx);
    A3 = Rbb(:, 3)' * dotx;
    D3 = -Rbb(:, 1)' * dotx;
    C3 = -Rbb(:, 2)' * g;
    if abs(A2*D3 - A3*D2) < 0.001
        wz = wz_;
        wx = (C2 - D2*wz)/A2;
        %wx = wx_;
        wy = (C1 - A1*wx - D1*wz)/B1;
        %disp('Omega Signarity')
    else
        wx = (C2*D3 - C3*D2)/(A2*D3 - A3*D2);
        wy = -(A1*C2*D3 - A1*C3*D2 - A2*C1*D3 + A2*C3*D1 + A3*C1*D2 - A3*C2*D1)/(B1*(A2*D3 - A3*D2));
        wz = (A2*C3 - A3*C2)/(A2*D3 - A3*D2);
        wz_ = wz;
        wx_ = wx;
    end
%     wx = -(D2*wsz - C2*cos(kk-alpha))/(A2*cos(kk-alpha) + D2*sin(kk-alpha));
%     wy = (A1*D2*wsz - A2*D1*wsz - A1*C2*cos(kk-alpha) + A2*C1*cos(kk-alpha) + C1*D2*sin(kk-alpha) - C2*D1*sin(kk-alpha))/(B1*(A2*cos(kk-alpha) + D2*sin(kk-alpha)));
%     wz = (A2*wsz + C2*sin(kk-alpha))/(A2*cos(kk-alpha) + D2*sin(kk-alpha));
    wbb = [wx; wy; wz];
    %wbb(2) = constrain(wbb(2), -3, 3); wbb(1) = constrain(wbb(1), -3, 3); wbb(3) = constrain(wbb(3), -3, 3);
end
